simulink model "QuadrotorModel"  (R2023b)
settings: Solver=VariableStepAuto  StartTime=0.0  StopTime=SimTime  RelTol=1e-3
values from neighbouring files (symbols this model uses):
  g = [g, {Xk_end - Xk}]    [Opitm_rizeni2.m]    (also in Quadcopter_simulace.m = 9.81; casadi_nmpc.m; drone_model2.m = 9.81)
  Ix = 1.395e-5    (= 1.395e-05)    [Quadcopter_simulace.m]    (also in casadi_nmpc.m; drone_model2.m)
  Iy = 1.436e-6    (= 1.436e-06)    [Quadcopter_simulace.m]    (also in casadi_nmpc.m; drone_model2.m)
  Iz = 2.173e-6    (= 2.173e-06)    [Quadcopter_simulace.m]    (also in casadi_nmpc.m; drone_model2.m)
  m = 0.03    [Quadcopter_simulace.m]    (also in casadi_nmpc.m; drone_model2.m)
libraries: matrix_library x1, aerolibutil x1, uavalgslib x1
settings Model: Creator=Ondra  LastModifiedBy=Ondra

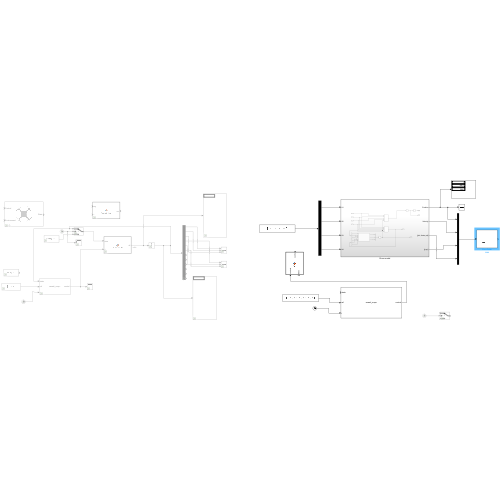
[thumbnail: Simulink's stored preview of the top-level diagram]
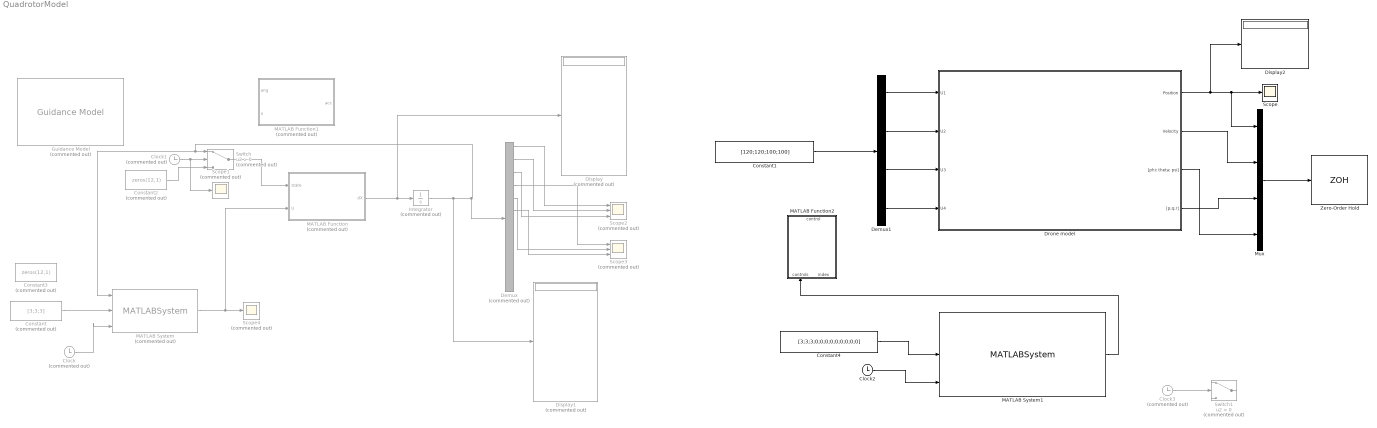
== system QuadrotorModel ==
  Clock : Clock  Commented=on
  Clock1 : Clock  Commented=on
  Clock2 : Clock
  Clock3 : Clock  Commented=on
  Constant : Constant  Commented=on  Value=[3;3;3]
  Constant1 : Constant  Value=[120;120;100;100]
  Constant2 : Constant  Commented=on  Value=zeros(12,1)
  Constant3 : Constant  Commented=on  Value=zeros(12,1)
  Constant4 : Constant  Value=[3;3;3;0;0;0;0;0;0;0;0;0]
  Demux : Demux  Commented=on  Outputs=12
  Demux1 : Demux
  Display : Display  Commented=on
  Display1 : Display  Commented=on
  Display2 : Display
  Drone model : Subsystem
  Guidance Model : uavalgslib/Guidance Model  Commented=on  ModelType=MultirotorGuidance  SpecifiedDataType=double  SimulateUsing=Interpreted execution  InitialWorldPositionMultirotor=[0; 0; 0]  InitialWorldVelocityMultirotor=[0; 0; 0]  InitialEulerZYXMultirotor=[0; 0; 0]  InitialBodyAngularRateRPYMultirotor=[0; 0; 0]  InitialThrustMultirotor=0  InitialNorthFixedWing=0  InitialEastFixedWing=0  InitialHeightFixedWing=0  InitialAirSpeedFixedWing=0  InitialHeadingAngleFixedWing=0  InitialFlightPathAngleFixedWing=0  InitialRollAngleFixedWing=0  InitialRollAngleRateFixedWing=0  PDRollMultirotor=[3402.97,116.67]  PDPitchMultirotor=[3402.97, 116.67]  PYawRateMultirotor=1950  PThrustMultirotor=3900  MassMultirotor=0.1  PHeightFixedWing=3.9  PHeadingAngleFixedWing=3.9  PFlightPathAngleFixedWing=39  PDRollFixedWing=[3402.97, 116.67]  PAirSpeedFixedWing=1  FlightPathAngleLimitsFixedWing=[-pi/2, pi/2]  StateBusName='MultirotorGuidanceStateBus'  ControlBusName='MultirotorGuidanceControlBus'  EnvironmentBusName='MultirotorGuidanceEnvironmentBus'  DataType=double
  Integrator : Integrator  Commented=on
  MATLAB Function : MATLAB Function  Commented=on  TreatAsAtomicUnit=on
  MATLAB Function1 : MATLAB Function  Commented=on  TreatAsAtomicUnit=on
  MATLAB Function2 : MATLAB Function  TreatAsAtomicUnit=on
  MATLAB System : MATLABSystem  Commented=on  System=casadi_nmpc  SimulateUsing=Interpreted execution
      mask Type: casadi_nmpc
      mask Display:
      | disp('casadi_nmpc');
      | port_label('input',1,'state');
      | port_label('input',2,'ref');
      | port_label('input',3,'t');
      | port_label('output',1,'control');
  MATLAB System1 : MATLABSystem  System=casadi_nmpc  SimulateUsing=Interpreted execution
      mask Type: casadi_nmpc
      mask Display:
      | disp('casadi_nmpc');
      | port_label('input',1,'state');
      | port_label('input',2,'ref');
      | port_label('input',3,'t');
      | port_label('output',1,'control');
  Mux : Mux
  Scope : Scope
  Scope1 : Scope  Commented=on
  Scope2 : Scope  Commented=on  NumInputPorts=3
  Scope3 : Scope  Commented=on  NumInputPorts=3
  Scope4 : Scope  Commented=on
  Switch : Switch  Commented=on  Criteria=u2 > Threshold  SaturateOnIntegerOverflow=off  InputSameDT=off
  Switch1 : Switch  Commented=on  Criteria=u2 > Threshold  SaturateOnIntegerOverflow=off  InputSameDT=off
  Zero-Order Hold : ZeroOrderHold  SampleTime=-1
  wires:
  MATLAB Function/1(dX) -> Display/1, Integrator/1
  Integrator/1 -> Display1/1, MATLAB System/1, Switch/1, Demux/1
  Constant/1 -> MATLAB System/2
  Clock/1 -> MATLAB System/3
  MATLAB System/1 -> MATLAB Function/2(U), Scope4/1
  Clock1/1 -> Scope1/1, Switch/2
  Demux/1 -> Scope2/1
  Demux/2 -> Scope2/2
  Demux/3 -> Scope2/3
  Demux/4 -> Scope3/1
  Demux/5 -> Scope3/2
  Demux/6 -> Scope3/3
  Switch/1 -> MATLAB Function/1(state)
  Constant2/1 -> Switch/3
  Demux1/1 -> Drone model/1(U1)
  Demux1/2 -> Drone model/2(U2)
  Demux1/3 -> Drone model/3(U3)
  Demux1/4 -> Drone model/4(U4)
  Drone model/1(Position) -> Display2/1, Mux/1, Scope/1
  Drone model/2(Velocity) -> Mux/2
  Drone model/4("[p;q;r]") -> Mux/3
  Drone model/3("[phi; theta; psi]") -> Mux/4
  Constant4/1 -> MATLAB System1/2
  Clock2/1 -> MATLAB System1/3
  MATLAB System1/1 -> MATLAB Function2/1(controls)
  Clock3/1 -> Switch1/2
  Constant1/1 -> Demux1/1
  Mux/1 -> Zero-Order Hold/1

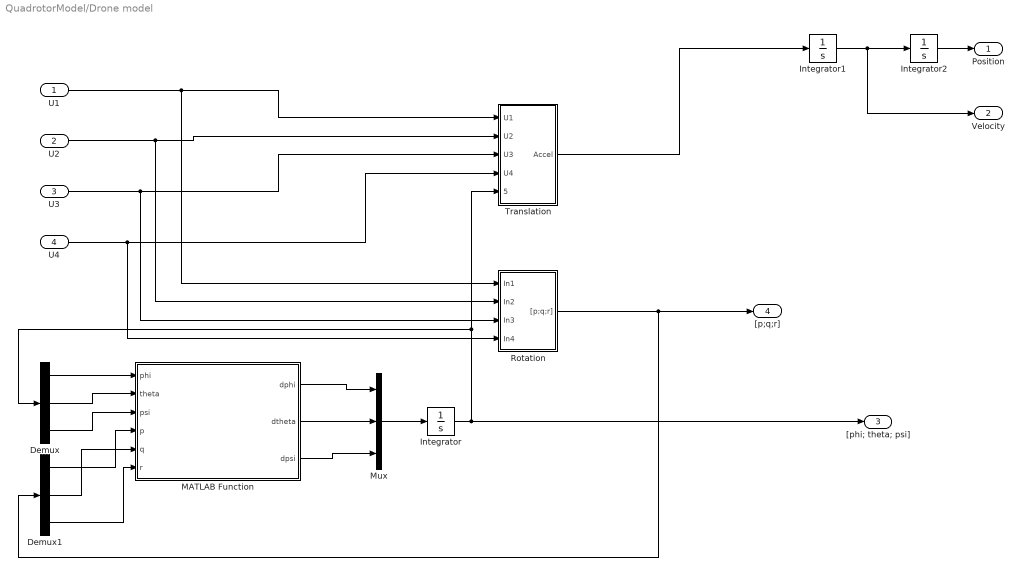
== system QuadrotorModel/Drone model ==
  U1 : Inport
  U2 : Inport  Port=2
  U3 : Inport  Port=3
  U4 : Inport  Port=4
  Demux : Demux  Outputs=3
  Demux1 : Demux  Outputs=3
  Integrator : Integrator
  Integrator1 : Integrator
  Integrator2 : Integrator
  MATLAB Function : MATLAB Function  TreatAsAtomicUnit=on
  Mux : Mux  Inputs=3
  Rotation : Subsystem
  Translation : Subsystem
  Position : Outport
  Velocity : Outport  Port=2
  "[phi; theta; psi]" : Outport  Port=3
  "[p;q;r]" : Outport  Port=4
  wires:
  U1/1 -> Rotation/1(In1), Translation/1(U1)
  U2/1 -> Rotation/2(In2), Translation/2(U2)
  U3/1 -> Rotation/3(In3), Translation/3(U3)
  U4/1 -> Rotation/4(In4), Translation/4(U4)
  Integrator/1 -> "[phi; theta; psi]"/1, Demux/1, Translation/5(Angles)
  Translation/1(Accel) -> Integrator1/1
  Integrator1/1 -> Velocity/1, Integrator2/1
  Rotation/1("[p;q;r]") -> "[p;q;r]"/1, Demux1/1
  Mux/1 -> Integrator/1
  MATLAB Function/1(dphi) -> Mux/1
  MATLAB Function/2(dtheta) -> Mux/2
  MATLAB Function/3(dpsi) -> Mux/3
  Demux/1 -> MATLAB Function/1(phi)
  Demux/2 -> MATLAB Function/2(theta)
  Demux/3 -> MATLAB Function/3(psi)
  Demux1/1 -> MATLAB Function/4(p)
  Demux1/2 -> MATLAB Function/5(q)
  Demux1/3 -> MATLAB Function/6(r)
  Integrator2/1 -> Position/1

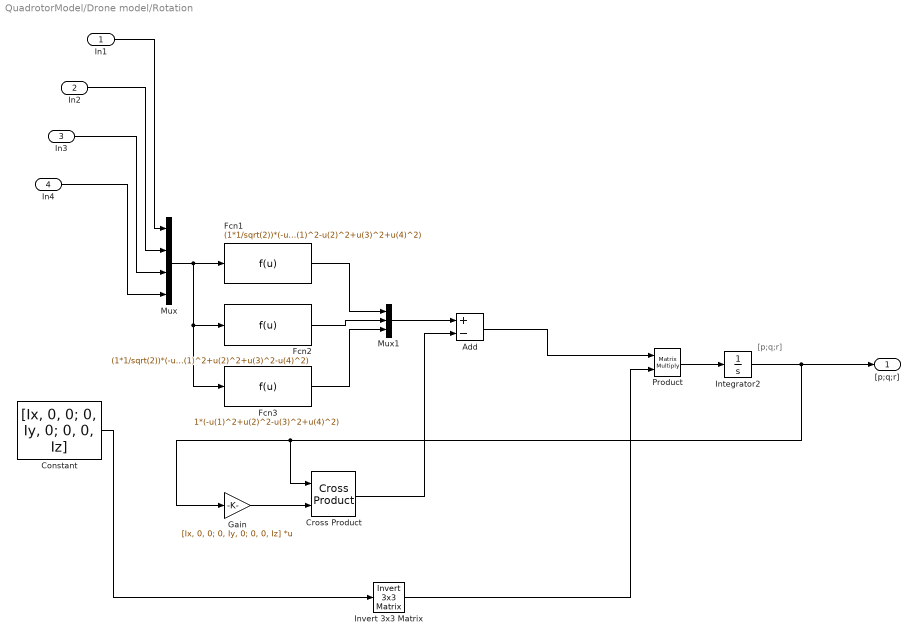
== system QuadrotorModel/Drone model/Rotation ==
  note: [p;q;r]
  In1 : Inport
  In2 : Inport  Port=2
  In3 : Inport  Port=3
  In4 : Inport  Port=4
  Add : Sum  Inputs=+-
  Constant : Constant  Value=[Ix, 0, 0; 0, Iy, 0; 0, 0, Iz]
  Cross Product : matrix_library/Cross Product
  Fcn1 : Fcn  Expr=(1*1/sqrt(2))*(-u(1)^2-u(2)^2+u(3)^2+u(4)^2)
  Fcn2 : Fcn  Expr=(1*1/sqrt(2))*(-u(1)^2+u(2)^2+u(3)^2-u(4)^2)
  Fcn3 : Fcn  Expr=1*(-u(1)^2+u(2)^2-u(3)^2+u(4)^2)
  Gain : Gain  Gain=[Ix, 0, 0; 0, Iy, 0; 0, 0, Iz]  Multiplication=Matrix(K*u) (u vector)
  Integrator2 : Integrator
  Invert 3x3 Matrix : aerolibutil/Invert  3x3 Matrix
  Mux : Mux
  Mux1 : Mux  Inputs=3
  Product : Product  Multiplication=Matrix(*)
  "[p;q;r]" : Outport
  wires:
  Constant/1 -> Invert 3x3 Matrix/1
  Cross Product/1 -> Add/2
  Mux/1 -> Fcn3/1, Fcn2/1, Fcn1/1
  Product/1 -> Integrator2/1
  Fcn2/1 -> Mux1/2
  Integrator2/1 -> "[p;q;r]"/1, Cross Product/1, Gain/1
  Fcn1/1 -> Mux1/1
  Add/1 -> Product/1
  In2/1 -> Mux/2
  Fcn3/1 -> Mux1/3
  Invert 3x3 Matrix/1 -> Product/2
  Mux1/1 -> Add/1
  In4/1 -> Mux/4
  In1/1 -> Mux/1
  In3/1 -> Mux/3
  Gain/1 -> Cross Product/2

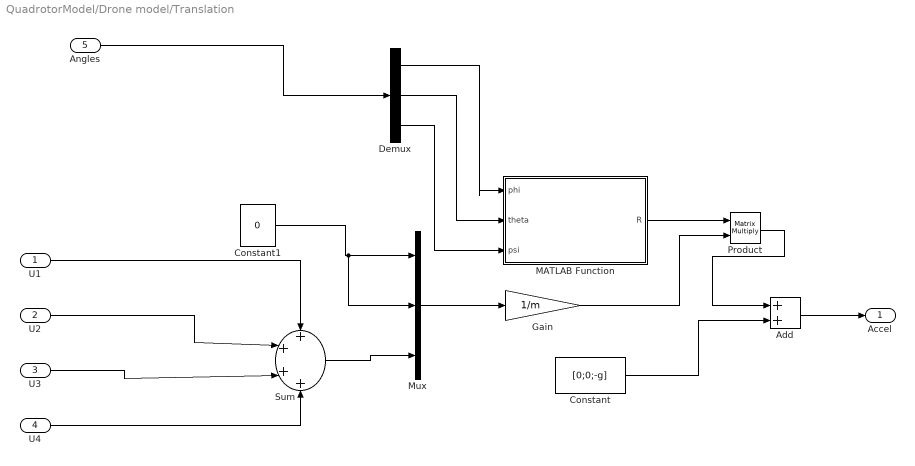
== system QuadrotorModel/Drone model/Translation ==
  U1 : Inport
  U2 : Inport  Port=2
  U3 : Inport  Port=3
  U4 : Inport  Port=4
  Angles : Inport  Port=5
  Add : Sum
  Constant : Constant  Value=[0;0;-g]
  Constant1 : Constant  Value=0
  Demux : Demux  Outputs=3
  Gain : Gain  Gain=1/m
  MATLAB Function : MATLAB Function  TreatAsAtomicUnit=on
  Mux : Mux  Inputs=3
  Product : Product  Multiplication=Matrix(*)
  Sum : Sum  Inputs=++++
  Accel : Outport
  wires:
  Demux/3 -> MATLAB Function/3(psi)
  Product/1 -> Add/1
  Demux/1 -> MATLAB Function/1(phi)
  U2/1 -> Sum/2
  Demux/2 -> MATLAB Function/2(theta)
  MATLAB Function/1(R) -> Product/1
  Constant/1 -> Add/2
  U3/1 -> Sum/3
  Angles/1 -> Demux/1
  U1/1 -> Sum/1
  U4/1 -> Sum/4
  Add/1 -> Accel/1
  Sum/1 -> Mux/3
  Constant1/1 -> Mux/2, Mux/1
  Mux/1 -> Gain/1
  Gain/1 -> Product/2

== matlab function QuadrotorModel/MATLAB Function1 ==
  data: ang input; acc output; u input
function acc = Translation(ang, u)
%ROT_MATRIX Summary of this function goes here
%   Detailed explanation goes here

g = 9.81;
phi = ang(1);
theta = ang(2);
psi = ang(3);
e3 = [0;0;3];
C_T = 1.28192e-8; % rotor thrust coefficient
m = 0.03;

% Rotace kolem osy Z (yaw)
R_psi = [cos(psi), -sin(psi), 0;
         sin(psi),  cos(psi), 0;
         0,        0,        1];
     
% Rotace kolem osy Y (pitch)
R_theta = [cos(theta), 0, sin(theta);
           0,          1, 0;
          -sin(theta), 0, cos(theta)];
      
% Rotace kolem osy X (roll)
R_phi = [1, 0,         0;
         0, cos(phi), -sin(phi);
         0, sin(phi),  cos(phi)];
     
% Celková rotační matice
Rot = R_psi * R_theta * R_phi;
Fz = C_T*sum(u.^2);
acc = -g*e3 + Rot*(Fz*e3)/m;    % [du;dv;dw]
end

== matlab function QuadrotorModel/MATLAB Function ==
  data: state input; dX output; U input
function dX = Drone_Model(state, U)
%ROT_MATRIX Summary of this function goes here
%   Detailed explanation goes here

%% Parametry
% kT = 3.16e-10; % rotor thrust coefficient
% ktau = 7.94e-12; % rotor torque coefficient
C_T = 1.28192e-8; % rotor thrust coefficient
C_M = 5.964552e-3; % rotor torque coefficient

rad_max = (2*pi*64*200)/60; % maximal angular rate of rotor [rad/s]
rad_min = (2*pi*64*18)/60; % minimal angular rate of rotor [rad/s]
rpm_max = rad_max*9.5492968;    % [rpm]
rpm_min = rad_min*9.5492968;    % [rpm]
arm_length = 0.0397; % arm length

g = 9.81; % gravitational acceleration
m = 0.03; % mass of quadrotor
m_lh = 0.032; % mass of quadrotor with lighthouse deck

% Ix = 2.3951e-5; % inertia of quadrotor around x-axis     
% Iy = 6.410179e-6; % inertia of quadrotor around y-axis
% Iz = 9.860228e-6; % inertia of quadrotor around z-axis
Ix = 1.395e-5; % inertia of quadrotor around x-axis     
Iy = 1.436e-6; % inertia of quadrotor around y-axis
Iz = 2.173e-6; % inertia of quadrotor around z-axis


Ts = 1e-3; % sampling period

% limit thrust
f_max = 0.15 * 4; % maximum collective thrust (single thrust f_i_max = 0.15)
f_min = 0.0;

% limit torque
tau_max = f_max * arm_length - f_min * arm_length;
tau_min = -tau_max;

% aerodynamic effect
K_aero = 1e-7 * [-10.2506, -0.3177, -0.4332;
                 -0.3177, -10.2506, -0.4332;
                 -7.7050, -7.7050, -7.5530];

u_stable = sqrt(g*m/(C_T*4));

%% Stavy
x = state(1); % pozice [x, y, z]
y = state(2);
z = state(3);
phi = state(4); % Eulerovy úhly [phi, theta, psi]
theta = state(5);
psi = state(6);
u = state(7); % rychlosti [vx, vy, vz]
v = state(8);
w = state(9);
p = state(10); % úhlové rychlosti [p, q, r]
q = state(11);
r = state(12);

%% Souradny system Zeme
E = eye(3);
e1 = E(:,1);
e2 = E(:,2);
e3 = E(:,3);

%% Rotacni matice
% Rotace kolem osy Z (yaw)
R_psi = [cos(psi), -sin(psi), 0;
         sin(psi),  cos(psi), 0;
         0,        0,        1];
     
% Rotace kolem osy Y (pitch)
R_theta = [cos(theta), 0, sin(theta);
           0,          1, 0;
          -sin(theta), 0, cos(theta)];
      
% Rotace kolem osy X (roll)
R_phi = [1, 0,         0;
         0, cos(phi), -sin(phi);
         0, sin(phi),  cos(phi)];
     
% Celková rotační matice
Rot = R_psi * R_theta * R_phi;
% Rot = [cos(theta), cos(theta)*sin(psi), -sin(theta);
%        sin(phi*sin(theta))*cos(psi)-cos(phi)*sin(psi), sin(phi*sin(theta))*sin(psi)+cos(phi)*cos(psi), sin(phi)*cos(theta);
%        cos(phi*sin(theta))*cos(psi)+sin(phi)*sin(psi), cos(phi*sin(theta))*sin(psi)-sin(phi)*cos(psi), cos(phi)*cos(theta)];

%% Translacni dynamika
Fz = C_T*sum(U.^2);
d_xyz = [u;v;w];
acc = -g*e3 + Rot*(Fz*e3)/m;    % [du;dv;dw]

%% Rotacni dynamika
J = diag([Ix, Iy, Iz]);
M = [(arm_length*C_T/sqrt(2))*(-U(1)^2-U(2)^2+U(3)^2+U(4)^2); ...
    (arm_length*C_T/sqrt(2))*(-U(1)^2+U(2)^2+U(3)^2-U(4)^2); ...
    C_M*(-U(1)^2+U(2)^2-U(3)^2+U(4)^2)];
ang_acc = inv(J)*(M - cross([p;q;r], J*[p;q;r]));

d_phi_theta_psi = [1, sin(phi)*tan(theta), cos(phi)*tan(theta);
                    0, cos(phi), -sin(phi);
                    0, sin(phi)/cos(theta), cos(phi)/cos(theta)]*[p;q;r];
%% Stavovy popis
dX = [d_xyz(1);
      d_xyz(2);
      d_xyz(3);
      acc(1);
      acc(2);
      acc(3);
      ang_acc(1);
      ang_acc(2);
      ang_acc(3);
      d_phi_theta_psi(1);
      d_phi_theta_psi(2);
      d_phi_theta_psi(3)
      ];
end

== matlab function QuadrotorModel/Drone model/Translation/MATLAB Function ==
  data: phi input; R output; theta input; psi input
function R = Rot_matrix(phi,theta, psi)
%ROT_MATRIX Summary of this function goes here
%   Detailed explanation goes here
% Rotace kolem osy Z (yaw)
R_psi = [cos(psi), -sin(psi), 0;
         sin(psi),  cos(psi), 0;
         0,        0,        1];
     
% Rotace kolem osy Y (pitch)
R_theta = [cos(theta), 0, sin(theta);
           0,          1, 0;
          -sin(theta), 0, cos(theta)];
      
% Rotace kolem osy X (roll)
R_phi = [1, 0,         0;
         0, cos(phi), -sin(phi);
         0, sin(phi),  cos(phi)];
     
% Celková rotační matice
R = R_psi * R_theta * R_phi;
end

== matlab function QuadrotorModel/Drone model/MATLAB Function ==
  data: phi input; dphi output; theta input; psi input; p input; q input; r input; dtheta output; dpsi output
function [dphi, dtheta, dpsi] = fcn(phi, theta, psi, p, q, r)
    d_phi_theta_psi = [1, sin(phi)*tan(theta), cos(phi)*tan(theta);
                       0, cos(phi), -sin(phi);
                       0, sin(phi)/cos(theta), cos(phi)/cos(theta)]*[p;q;r];

dphi = d_phi_theta_psi(1);
dtheta = d_phi_theta_psi(2);
dpsi = d_phi_theta_psi(3);

== matlab function QuadrotorModel/MATLAB Function2 ==
  data: controls input; control output; index input
function control = fcn(controls, index)

control = controls(index);
